simulink model "PCCM_RPU_Interface"  (R2016b)
settings: Solver=FixedStepDiscrete  StartTime=0.0  StopTime=inf  FixedStep=PCCMRPUIf.tiSimnTiStep_C  RelTol=1e-3  EnableMultiTasking=on
settings Model: Creator=m01wolf  LastModifiedBy=sevren
settings DataIOCC: SaveFormat=StructureWithTime  SaveOutput=off  DSMLogging=off  VisualizeSimOutput=off  SaveTime=off  StateSaveName=Results  SignalLoggingName=Results
settings OptimizationCC: BlockReduction=off  ConditionallyExecuteInputs=off  LifeSpan=inf
settings DebuggingCC: AllowSymbolicDim=off  SFUnexpectedBacktrackingDiag=warning  SFNoUnconditionalDefaultTransitionDiag=warning  SFExecutionAtInitializationDiag=none
settings ModelReferenceCC: ModelReferenceNumInstancesAllowed=Single  PropagateSignalLabelsOutOfModel=off
settings GRTTargetCC: TargetLangStandard=C89/C90 (ANSI)
settings ConfigComp: CovMetricSettings=dw  CovHtmlReporting=on  CovSaveCumulativeToWorkspaceVar=on  CovSaveSingleToWorkspaceVar=on  CovExternalEMLEnable=off

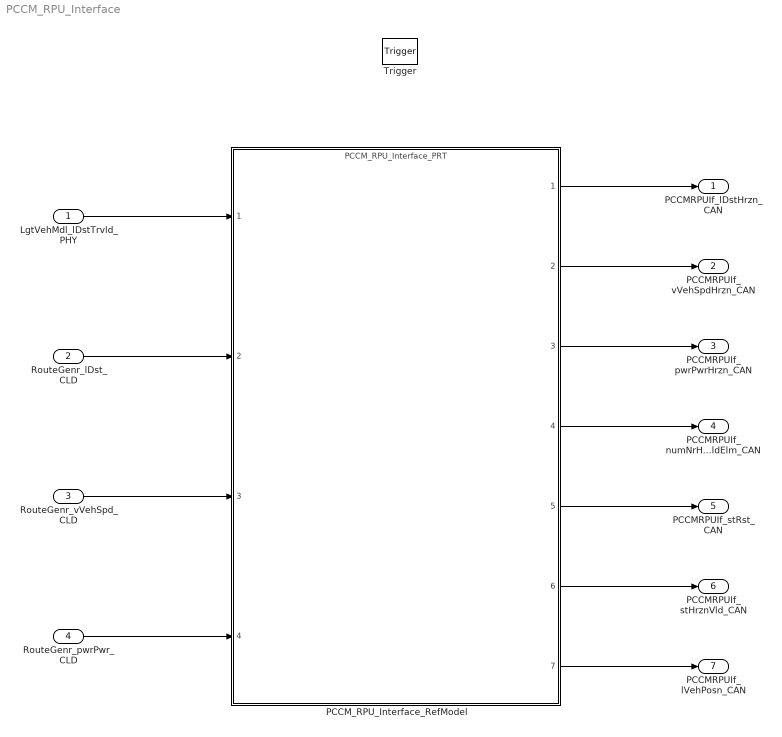
== system PCCM_RPU_Interface ==
  LgtVehMdl_lDstTrvld_PHY : Inport
  RouteGenr_lDst_CLD : Inport  Port=2
  RouteGenr_vVehSpd_CLD : Inport  Port=3
  RouteGenr_pwrPwr_CLD : Inport  Port=4
  Trigger : TriggerPort  TriggerType=function-call  VariantControl=Variant  PortDimensions=1
  PCCM_RPU_Interface_RefModel : ModelReference  ModelNameDialog=PCCM_RPU_Interface_PRT.slxp  ModelReferenceVersion=1.255  CopyOfModelProtected=on
  PCCMRPUIf_lDstHrzn_CAN : Outport
  PCCMRPUIf_vVehSpdHrzn_CAN : Outport  Port=2
  PCCMRPUIf_pwrPwrHrzn_CAN : Outport  Port=3
  PCCMRPUIf_numNrHrznVldElm_CAN : Outport  Port=4
  PCCMRPUIf_stRst_CAN : Outport  Port=5
  PCCMRPUIf_stHrznVld_CAN : Outport  Port=6
  PCCMRPUIf_lVehPosn_CAN : Outport  Port=7
  wires:
  PCCM_RPU_Interface_RefModel/1 -> PCCMRPUIf_lDstHrzn_CAN/1
  PCCM_RPU_Interface_RefModel/7 -> PCCMRPUIf_lVehPosn_CAN/1
  PCCM_RPU_Interface_RefModel/3 -> PCCMRPUIf_pwrPwrHrzn_CAN/1
  PCCM_RPU_Interface_RefModel/2 -> PCCMRPUIf_vVehSpdHrzn_CAN/1
  PCCM_RPU_Interface_RefModel/4 -> PCCMRPUIf_numNrHrznVldElm_CAN/1
  PCCM_RPU_Interface_RefModel/5 -> PCCMRPUIf_stRst_CAN/1
  PCCM_RPU_Interface_RefModel/6 -> PCCMRPUIf_stHrznVld_CAN/1
  LgtVehMdl_lDstTrvld_PHY/1 -> PCCM_RPU_Interface_RefModel/1
  RouteGenr_lDst_CLD/1 -> PCCM_RPU_Interface_RefModel/2
  RouteGenr_vVehSpd_CLD/1 -> PCCM_RPU_Interface_RefModel/3
  RouteGenr_pwrPwr_CLD/1 -> PCCM_RPU_Interface_RefModel/4
